simulink model "PV_modelleme"  (R2018a)
settings: Solver=VariableStepAuto  StartTime=0.0  StopTime=4  RelTol=1e-3  AbsTol=1e-3  EnableMultiTasking=on
values from neighbouring files (symbols this model uses):
  n = n+1    (= 1)    [LVQ_kodu.m]    (also in MLNN1_kodu.m; MLNN2_kodu.m; pnn_kodu.m)
undefined symbols (not defined in the file or in its folder): Eg0, K, q, Tn
libraries: simulink x3
settings Model: Creator=Tolga  LastModifiedBy=Tolga
settings SolverCC: AutoScaleAbsTol=off
settings DataIOCC: LimitDataPoints=on  MaxDataPoints=10000
settings OptimizationCC: LifeSpan=inf
settings DebuggingCC: AllowSymbolicDim=off  SFUnexpectedBacktrackingDiag=warning  SFNoUnconditionalDefaultTransitionDiag=warning  SFExecutionAtInitializationDiag=none
settings CodeAppCC: StateflowObjectComments=on
settings GRTTargetCC: TargetLangStandard=C89/C90 (ANSI)  GeneratePreprocessorConditionals=Disable all
settings ConfigComp: CovMetricSettings=dw  CovHtmlReporting=on  CovSaveCumulativeToWorkspaceVar=on  CovSaveSingleToWorkspaceVar=on  CovExternalEMLEnable=off  CovSFcnEnable=off
settings SimscapeCC: SimscapeLogType=all  SimscapeLogDataHistory=10000

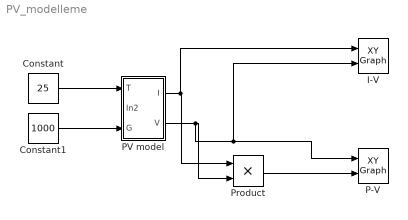
== system PV_modelleme ==
  Constant : Constant  Value=25
  Constant1 : Constant  Value=1000
  "I-V " : simulink/Sinks/XY Graph  xmin=0  xmax=35  ymin=0  ymax=10  st=-1
  P-V : simulink/Sinks/XY Graph  xmin=0  xmax=35  ymin=0  ymax=210  st=-1
  PV model : Subsystem  InitFcn=|
      | ki=.0032,
      | q=1.6e-19,
      | K=1.38e-23,
      | n=1.3,
      | Eg0=1.1,
      | Rs=.221,
      | Rsh=415.405,
      | Tn=298,
      | 
      | Voc=32.9,
      | Isc=8.21,
      | Ns=54,
  Product : Product
  wires:
  Constant1/1 -> PV model/3(G)
  Constant/1 -> PV model/1(T)
  Product/1 -> P-V/2
  PV model/2(V) -> "I-V "/2, P-V/1, Product/2
  PV model/1(I) -> "I-V "/1, Product/1

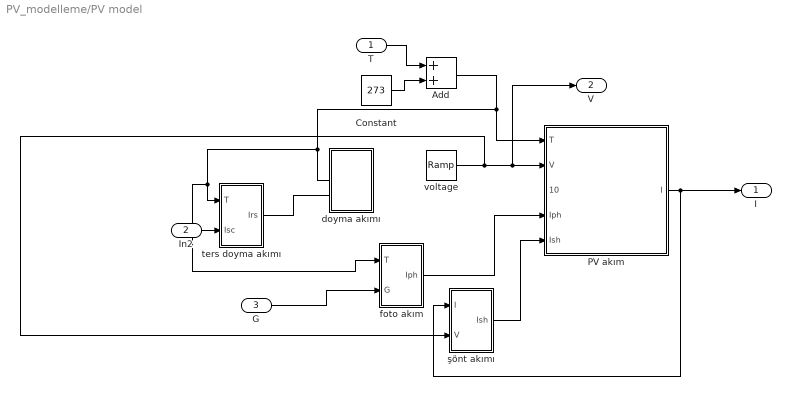
== system PV_modelleme/PV model ==
  T : Inport
  In2 : Inport  Port=2
  G : Inport  Port=3
  Add : Sum
  Constant : Constant  Value=273
  PV akım : Subsystem
  doyma akımı : Subsystem
  foto akım : Subsystem
  ters doyma akımı : Subsystem
  voltage : simulink/Sources/Ramp  slope=10  start=0  InitialOutput=0
  şönt akımı : Subsystem
  I : Outport
  V : Outport  Port=2
  wires:
  ters doyma akımı/1(Irs) -> ?
  PV akım/1(I) -> I/1, şönt akımı/1("I ")
  G/1 -> foto akım/2(G)
  voltage/1 -> şönt akımı/2("V "), V/1, PV akım/2(V)
  Add/1 -> foto akım/1(T), ters doyma akımı/1(T), PV akım/1(T)
  Constant/1 -> Add/2
  ? -> PV akım/3(10)
  foto akım/1(Iph) -> PV akım/4(Iph)
  şönt akımı/1(Ish) -> PV akım/5(Ish)
  T/1 -> Add/1
  In2/1 -> ters doyma akımı/2(Isc)

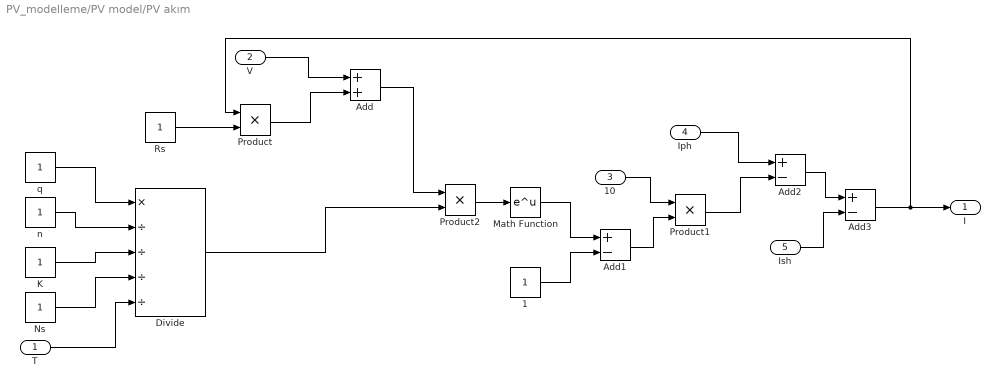
== system PV_modelleme/PV model/PV akım ==
  T : Inport
  V : Inport  Port=2
  10 : Inport  Port=3
  Iph : Inport  Port=4
  Ish : Inport  Port=5
  1 : Constant
  Add : Sum
  Add1 : Sum  Inputs=+-
  Add2 : Sum  Inputs=+-
  Add3 : Sum  Inputs=+-
  Divide : Product  Inputs=*////
  K : Constant
  Math Function : Math  SaturateOnIntegerOverflow=on
  Ns : Constant
  Product : Product
  Product1 : Product
  Product2 : Product
  Rs : Constant
  n : Constant
  q : Constant
  I : Outport
  wires:
  n/1 -> Divide/2
  Product/1 -> Add/2
  Add/1 -> Product2/1
  Add3/1 -> I/1, Product/1
  Math Function/1 -> Add1/1
  Product2/1 -> Math Function/1
  10/1 -> Product1/1
  K/1 -> Divide/3
  1/1 -> Add1/2
  Ns/1 -> Divide/4
  T/1 -> Divide/5
  Divide/1 -> Product2/2
  q/1 -> Divide/1
  Rs/1 -> Product/2
  Product1/1 -> Add2/2
  Add2/1 -> Add3/1
  V/1 -> Add/1
  Add1/1 -> Product1/2
  Iph/1 -> Add2/1
  Ish/1 -> Add3/2

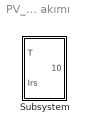
== system PV_modelleme/PV model/doyma akımı ==
  Subsystem : Subsystem

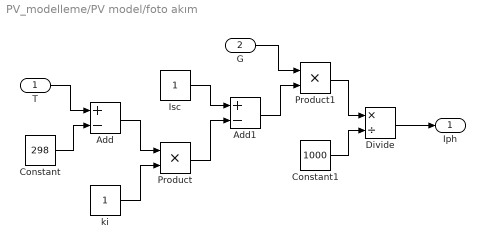
== system PV_modelleme/PV model/foto akım ==
  T : Inport
  G : Inport  Port=2
  Add : Sum  Inputs=+-
  Add1 : Sum  Inputs=+-
  Constant : Constant  Value=298
  Constant1 : Constant  Value=1000
  Divide : Product  Inputs=*/
  Isc : Constant
  Product : Product
  Product1 : Product
  ki : Constant
  Iph : Outport
  wires:
  Product/1 -> Add1/2
  ki/1 -> Product/2
  G/1 -> Product1/1
  Add/1 -> Product/1
  Divide/1 -> Iph/1
  Isc/1 -> Add1/1
  Constant1/1 -> Divide/2
  Constant/1 -> Add/2
  T/1 -> Add/1
  Add1/1 -> Product1/2
  Product1/1 -> Divide/1

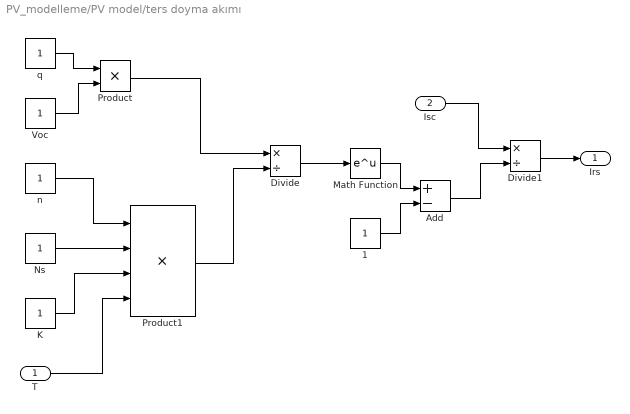
== system PV_modelleme/PV model/ters doyma akımı ==
  T : Inport
  Isc : Inport  Port=2
  1 : Constant
  Add : Sum  Inputs=+-
  Divide : Product  Inputs=*/
  Divide1 : Product  Inputs=*/
  K : Constant
  Math Function : Math  SaturateOnIntegerOverflow=on
  Ns : Constant
  Product : Product
  Product1 : Product  Inputs=4
  Voc : Constant
  n : Constant
  q : Constant
  Irs : Outport
  wires:
  1/1 -> Add/2
  T/1 -> Product1/4
  Isc/1 -> Divide1/1
  K/1 -> Product1/3
  Product1/1 -> Divide/2
  Ns/1 -> Product1/2
  Product/1 -> Divide/1
  Add/1 -> Divide1/2
  q/1 -> Product/1
  Divide1/1 -> Irs/1
  Divide/1 -> Math Function/1
  Math Function/1 -> Add/1
  n/1 -> Product1/1
  Voc/1 -> Product/2

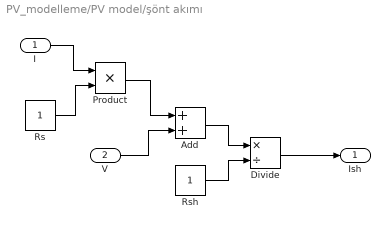
== system PV_modelleme/PV model/şönt akımı ==
  "I " : Inport
  "V " : Inport  Port=2
  Add : Sum
  Divide : Product  Inputs=*/
  Product : Product
  Rs : Constant
  Rsh : Constant
  Ish : Outport
  wires:
  Add/1 -> Divide/1
  "I "/1 -> Product/1
  Divide/1 -> Ish/1
  Product/1 -> Add/1
  Rsh/1 -> Divide/2
  Rs/1 -> Product/2
  "V "/1 -> Add/2

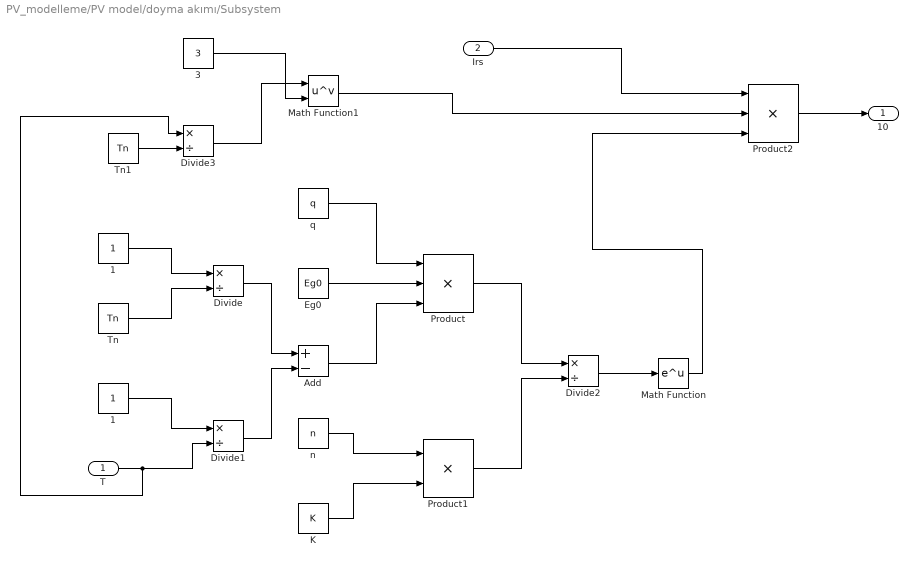
== system PV_modelleme/PV model/doyma akımı/Subsystem ==
  T : Inport
  Irs : Inport  Port=2
  1 : Constant
  "1 " : Constant
  3 : Constant  Value=3
  Add : Sum  Inputs=+-
  Divide{,1..3} (4 alike) : Product  Inputs=*/
  Eg0 : Constant  Value=Eg0
  K : Constant  Value=K
  Math Function : Math  SaturateOnIntegerOverflow=on
  Math Function1 : Math  Operator=pow  SaturateOnIntegerOverflow=on
  Product : Product  Inputs=3
  Product1 : Product
  Product2 : Product  Inputs=3
  Tn : Constant  Value=Tn
  Tn1 : Constant  Value=Tn
  n : Constant  Value=n
  q : Constant  Value=q
  10 : Outport
  wires:
  Eg0/1 -> Product/2
  Tn1/1 -> Divide3/2
  Divide2/1 -> Math Function/1
  3/1 -> Math Function1/2
  Product/1 -> Divide2/1
  Divide1/1 -> Add/2
  1/1 -> Divide1/1
  Add/1 -> Product/3
  Irs/1 -> Product2/1
  Tn/1 -> Divide/2
  Divide3/1 -> Math Function1/1
  Math Function/1 -> Product2/3
  Product1/1 -> Divide2/2
  Divide/1 -> Add/1
  T/1 -> Divide1/2, Divide3/1
  n/1 -> Product1/1
  Product2/1 -> 10/1
  q/1 -> Product/1
  K/1 -> Product1/2
  "1 "/1 -> Divide/1
  Math Function1/1 -> Product2/2
